simulink model "vozidla4_discrete"  (R2021a)
settings: Solver=VariableStepAuto  StartTime=0.0  StopTime=100  RelTol=1e-3
values from neighbouring files (symbols this model uses):
  conds = zeros(1,numOfStates)    [hl_script_rozsireniBP.m]
  Cw = Cw1    [hl_script_rozsireniBP.m]
  Cy = zeros(N,numOfStates)    [systemGen.m]
  eigenvals = [p q r]    [hl_script_rozsireniBP.m]
  inputDist = 1    [hl_script_rozsireniBP.m]
  Kdb = [-0.5820    0.0000   -0.0000    0.0000    0.0000    0.0000   -0.0000 ... (first row only)    [hl_script_rozsireniBP.m]
  setpoints = zeros(numOfStates,1)    [hl_script_rozsireniBP.m]
  structure = 5    [hl_script_rozsireniBP.m]
  sysD = c2d(sysC,Ts,'zoh')    [hl_script_rozsireniBP.m]
  Ts = 1    [hl_script_rozsireniBP.m]
libraries: simulink x1
settings Model: Creator=radek  LastModifiedBy=radek

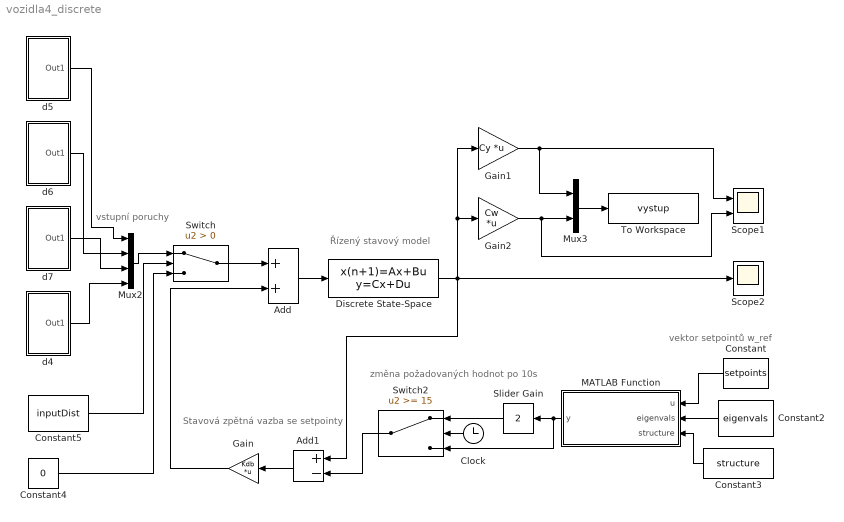
== system vozidla4_discrete ==
  note: vektor setpointů w_ref
  note: změna požadovaných hodnot po 10s
  note: vstupní poruchy
  note: Řízený stavový model
  note: Stavová zpětná vazba se setpointy
  Add : Sum
  Add1 : Sum  Inputs=+-
  Clock : Clock
  Constant : Constant  Value=setpoints
  Constant2 : Constant  Value=eigenvals
  Constant3 : Constant  Value=structure
  Constant4 : Constant  Value=0  SampleTime=Ts
  Constant5 : Constant  Value=inputDist  SampleTime=Ts
  Discrete State-Space : DiscreteStateSpace  A=sysD.A  B=sysD.B  C=sysD.C  D=sysD.D  InitialCondition=conds  SampleTime=Ts
  Gain : Gain  Gain=Kdb  Multiplication=Matrix(K*u)
  Gain1 : Gain  Gain=Cy  Multiplication=Matrix(K*u)
  Gain2 : Gain  Gain=Cw  Multiplication=Matrix(K*u)
  MATLAB Function : MATLAB Function  TreatAsAtomicUnit=on
  Mux2 : Mux
  Mux3 : Mux  Inputs=2
  Scope1 : Scope  NumInputPorts=2
  Scope2 : Scope
  Slider Gain : simulink/Math Operations/Slider Gain  gain=2  low=0  high=4
  Switch : Switch  Criteria=u2 > Threshold
  Switch2 : Switch  Threshold=15
  To Workspace : ToWorkspace  VariableName=vystup  SaveFormat=Structure  SampleTime=Ts
  d4 : Subsystem
  d5 : Subsystem
  d6 : Subsystem
  d7 : Subsystem
  wires:
  d4/1(Out1) -> Mux2/4
  Switch2/1 -> Add1/2
  Add/1 -> Discrete State-Space/1
  Discrete State-Space/1 -> Add1/1, Scope2/1, Gain1/1, Gain2/1
  d7/1(Out1) -> Mux2/3
  Constant3/1 -> MATLAB Function/3(structure)
  d5/1(Out1) -> Mux2/1
  Gain/1 -> Add/2
  Mux2/1 -> Switch/1
  Constant/1 -> MATLAB Function/1(u)
  d6/1(Out1) -> Mux2/2
  Slider Gain/1 -> Switch2/1
  Switch/1 -> Add/1
  Gain2/1 -> Scope1/2, Mux3/2
  MATLAB Function/1(y) -> Switch2/3, Slider Gain/1
  Constant2/1 -> MATLAB Function/2(eigenvals)
  Gain1/1 -> Scope1/1, Mux3/1
  Constant5/1 -> Switch/2
  Constant4/1 -> Switch/3
  Add1/1 -> Gain/1
  Clock/1 -> Switch2/2
  Mux3/1 -> To Workspace/1

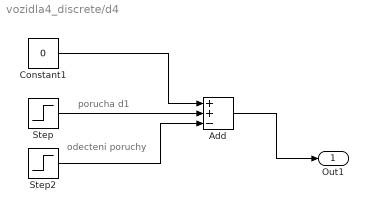
== system vozidla4_discrete/d4 ==
  note: odecteni poruchy
  note: porucha d1
  Add : Sum  Inputs=++-
  Constant1 : Constant  Value=0  SampleTime=Ts
  Step : Step  Time=65  After=2  SampleTime=Ts
  Step2 : Step  Time=66  After=2  SampleTime=Ts
  Out1 : Outport
  wires:
  Constant1/1 -> Add/1
  Step2/1 -> Add/3
  Add/1 -> Out1/1
  Step/1 -> Add/2

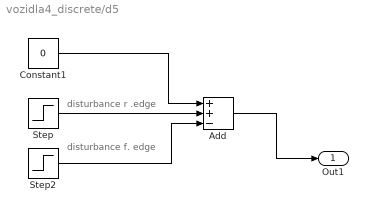
== system vozidla4_discrete/d5 ==
  note: disturbance f. edge
  note: disturbance r .edge
  Add : Sum  Inputs=++-
  Constant1 : Constant  Value=0  SampleTime=Ts
  Step : Step  Time=5  After=2  SampleTime=Ts
  Step2 : Step  Time=6  After=2  SampleTime=Ts
  Out1 : Outport
  wires:
  Constant1/1 -> Add/1
  Add/1 -> Out1/1
  Step/1 -> Add/2
  Step2/1 -> Add/3

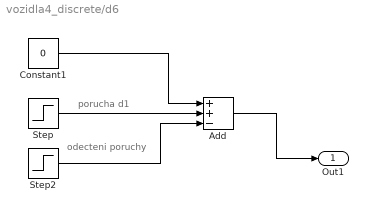
== system vozidla4_discrete/d6 ==
  note: odecteni poruchy
  note: porucha d1
  Add : Sum  Inputs=++-
  Constant1 : Constant  Value=0  SampleTime=Ts
  Step : Step  Time=25  After=2  SampleTime=Ts
  Step2 : Step  Time=26  After=2  SampleTime=Ts
  Out1 : Outport
  wires:
  Constant1/1 -> Add/1
  Step2/1 -> Add/3
  Add/1 -> Out1/1
  Step/1 -> Add/2

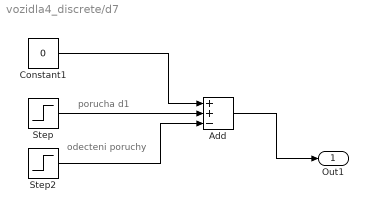
== system vozidla4_discrete/d7 ==
  note: odecteni poruchy
  note: porucha d1
  Add : Sum  Inputs=++-
  Constant1 : Constant  Value=0
  Step : Step  Time=45  After=2  SampleTime=Ts
  Step2 : Step  Time=46  After=2  SampleTime=Ts
  Out1 : Outport
  wires:
  Constant1/1 -> Add/1
  Step2/1 -> Add/3
  Add/1 -> Out1/1
  Step/1 -> Add/2

== matlab function vozidla4_discrete/MATLAB Function ==
  data: u input; y output; eigenvals input; structure input
function y = Pgain(u,eigenvals,structure)
lambda = eigenvals(1);
nu = eigenvals(2);
if structure == 1
    temp = lambda/(lambda-1);
elseif structure == 2  
    temp = nu/(nu-1);
elseif structure == 3
    if lambda == nu
        temp = (lambda+nu)/(lambda+nu-2);
    else
        temp = lambda/(lambda-1);
    end
elseif structure == 5
    % lqr
    if eigenvals(3) == 1
        temp = (eigenvals(1)+1)/(eigenvals(1));
    else
        temp = (eigenvals(1)+1)/eigenvals(3);
% temp = 1;
    end
else
    temp = 1;
end
u(1:2:length(u)) = u(1:2:length(u))*temp;
y = u;
